simulink model "SimSILCase2"  (R2021b)
settings: Solver=VariableStepAuto  StartTime=0.0  StopTime=10.0  RelTol=1e-3
model workspace (MAT data in the model file):
  ConnVar.ipAddress = '192.168.0.153'
  ConnVar.user = ''
  ConnVar.pwd = []
  ConnVar.targetHandle = 0
undefined symbols (not defined in the file or in its folder): Comm
libraries: M1SWBlocks x3
settings Model: Creator=ebnicher  LastModifiedBy=gione

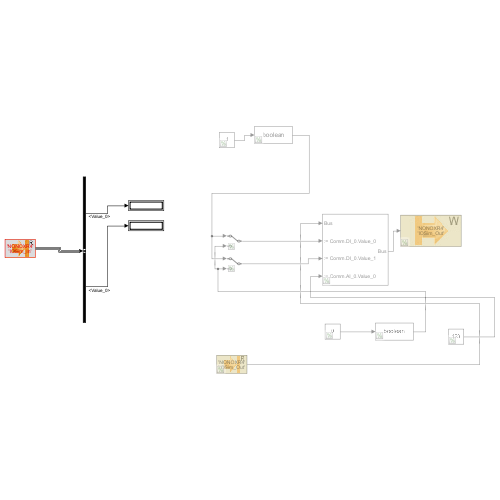
[thumbnail: Simulink's stored preview of the top-level diagram]
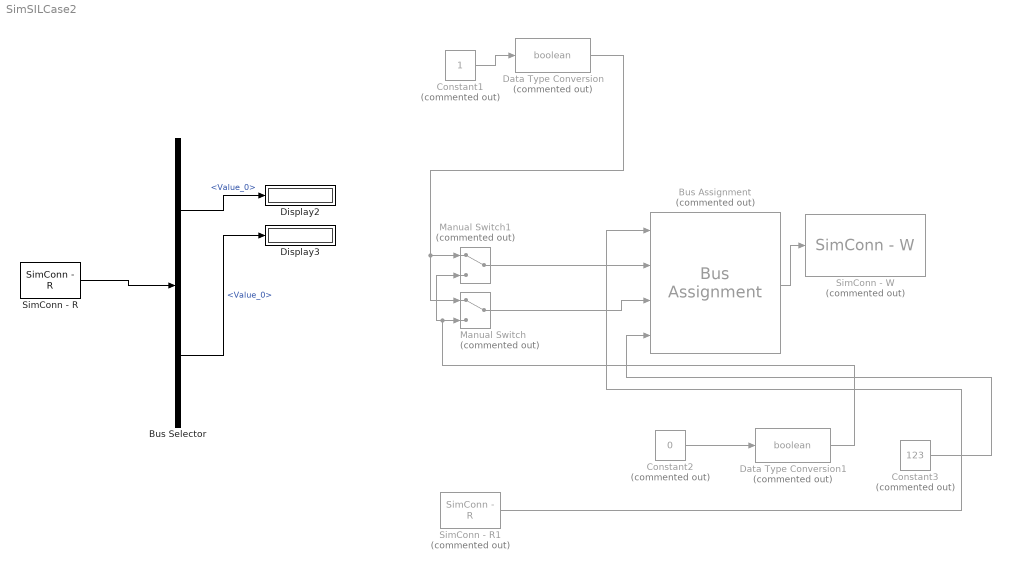
== system SimSILCase2 ==
  Bus Assignment : BusAssignment  Commented=on  AssignedSignals=Comm.DI_0.Value_0,Comm.DI_0.Value_1,Comm.AI_0.Value_0
  Bus Selector : BusSelector  OutputSignals=Comm.DO_0.Value_0,Comm.AO_0.Value_0
  Constant1 : Constant  Commented=on
  Constant2 : Constant  Commented=on  Value=0
  Constant3 : Constant  Commented=on  Value=123
  Data Type Conversion : DataTypeConversion  Commented=on  OutDataTypeStr=boolean
  Data Type Conversion1 : DataTypeConversion  Commented=on  OutDataTypeStr=boolean
  Display2 : Display
  Display3 : Display
  Manual Switch : ManualSwitch  Commented=on
  Manual Switch1 : ManualSwitch  Commented=on
  SimConn - R : M1SWBlocks/SimConn Blocks/SimConn - R  connVarName=ConnVar  InswModuleName='NONOXR4'  swModuleName=NONOXR4  InvarName='IOSim_In'  varName=IOSim_In  varDataType=Bus: IOSimIn  enRetOutput=off  enGetTrigger=off  getTrigger=rising  valDurLostConn=Zero  internalVal=0  DataDim=1  enSampTimMon=off  sampleTime=1
      settings: SourceProductName=Bachmann M1 Software
  SimConn - R1 : M1SWBlocks/SimConn Blocks/SimConn - R  Commented=on  connVarName=ConnVar  InswModuleName='NONOXR4'  swModuleName=NONOXR4  InvarName='IOSim_Out'  varName=IOSim_Out  varDataType=Bus: IOSimOut  enRetOutput=off  enGetTrigger=off  getTrigger=rising  valDurLostConn=Zero  internalVal=0  DataDim=1  enSampTimMon=off  sampleTime=1
      settings: SourceProductName=Bachmann M1 Software
  SimConn - W : M1SWBlocks/SimConn Blocks/SimConn - W  Commented=on  connVarName=ConnVar  InswModuleName='NONOXR4'  swModuleName=NONOXR4  InvarName='IOSim_Out'  varName=IOSim_Out  varDataType=Bus: IOSimOut  enRetOutput=off  enGetTrigger=off  getTrigger=rising  enSampTimMon=off
      settings: SourceProductName=Bachmann M1 Software
  wires:
  SimConn - R/1 -> Bus Selector/1
  Bus Selector/1 -> Display2/1  "<Value_0>"
  Bus Selector/2 -> Display3/1  "<Value_0>"
  Manual Switch1/1 -> Bus Assignment/2
  Manual Switch/1 -> Bus Assignment/3
  Data Type Conversion/1 -> Manual Switch/1, Manual Switch1/1
  Data Type Conversion1/1 -> Manual Switch/2, Manual Switch1/2
  SimConn - R1/1 -> Bus Assignment/1
  Bus Assignment/1 -> SimConn - W/1
  Constant3/1 -> Bus Assignment/4
  Constant1/1 -> Data Type Conversion/1
  Constant2/1 -> Data Type Conversion1/1
